simulink model "SUBSISTEMA_1"  (R2024b)
settings: Solver=VariableStepAuto  StartTime=0.0  StopTime=10.0  RelTol=1e-3
settings Model: Creator=juani  LastModifiedBy=juani

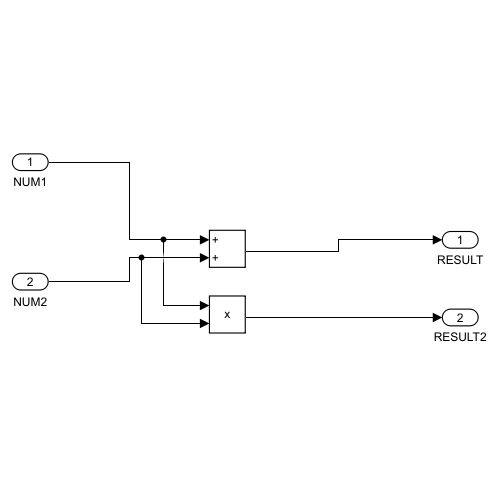
[thumbnail: Simulink's stored preview of the top-level diagram]
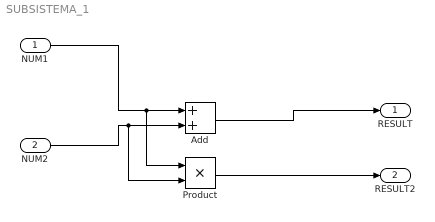
== system SUBSISTEMA_1 ==
  NUM1 : Inport
  NUM2 : Inport  Port=2
  Add : Sum
  Product : Product
  RESULT : Outport
  RESULT2 : Outport  Port=2
  wires:
  NUM1/1 -> Product/1, Add/1
  NUM2/1 -> Product/2, Add/2
  Add/1 -> RESULT/1
  Product/1 -> RESULT2/1
